simulink model "final_dynamic_24a"  (R2025a)
settings: Solver=ode15s  StartTime=0.0  StopTime=14000  RelTol=1e-3  AbsTol=1e-6
undefined symbols (not defined in the file): A_rad, bp_er, bp_mf, bp_speed, Cp_rad, epsilon, ETAT_table, h_h, M_rad, m_ratio_bp, mdot_design, paper54, PR_table, speed_bp, table_eff, table_mf, theta
libraries: simulink x4
(part 2 of 2)

== system final_dynamic_24a/rediator/Subsystem ==
  Constant : Constant  Value=epsilon
  Constant1 : Constant  Value=theta
  Constant2 : Constant  Value=A_rad
  Constant3 : Constant  Value=M_rad
  Constant4 : Constant  Value=Cp_rad
  Constant5 : Constant  Value=h_h
  epsilon : Outport
  theta : Outport  Port=2
  A_rad : Outport  Port=3
  M_rad : Outport  Port=4
  Cp_rad : Outport  Port=5
  h_h : Outport  Port=6
  wires:
  Constant3/1 -> M_rad/1
  Constant5/1 -> h_h/1
  Constant2/1 -> A_rad/1
  Constant1/1 -> theta/1
  Constant/1 -> epsilon/1
  Constant4/1 -> Cp_rad/1

== system final_dynamic_24a/TAC/Compressor/Corrected_Coordinates ==
  N_rpm : Inport
  mdot : Inport  Port=2
  P_in : Inport  Port=3
  T_in : Inport  Port=4
  CorrectedFlow : Product  Inputs=**/
  CorrectedSpeed : Product  Inputs=*/
  FlowAboveMinimum : simulink/Logic and Bit Operations/Compare To Constant  relop=>=  const=m_ratio_bp(1)  OutDataTypeStr=boolean
  FlowAboveMinimum_Assertion : Assertion
  FlowBelowMaximum : simulink/Logic and Bit Operations/Compare To Constant  relop=<=  const=m_ratio_bp(end)  OutDataTypeStr=boolean
  FlowBelowMaximum_Assertion : Assertion
  N_over_Ndesign : Gain  Gain=1/paper54.N_rpm
  P_over_Pdesign : Gain  Gain=1/paper54.compressor.Pin_Pa
  SpeedAboveMinimum : simulink/Logic and Bit Operations/Compare To Constant  relop=>=  const=speed_bp(1)  OutDataTypeStr=boolean
  SpeedAboveMinimum_Assertion : Assertion
  SpeedBelowMaximum : simulink/Logic and Bit Operations/Compare To Constant  relop=<=  const=speed_bp(end)  OutDataTypeStr=boolean
  SpeedBelowMaximum_Assertion : Assertion
  T_over_Tdesign : Gain  Gain=1/paper54.compressor.Tin_K
  mdot_over_mdesign : Gain  Gain=1/mdot_design
  sqrt_T_ratio : Math  Operator=sqrt
  speed_ratio : Outport
  flow_ratio : Outport  Port=2
  wires:
  SpeedAboveMinimum/1 -> SpeedAboveMinimum_Assertion/1
  SpeedBelowMaximum/1 -> SpeedBelowMaximum_Assertion/1
  FlowAboveMinimum/1 -> FlowAboveMinimum_Assertion/1
  FlowBelowMaximum/1 -> FlowBelowMaximum_Assertion/1
  N_rpm/1 -> N_over_Ndesign/1
  mdot/1 -> mdot_over_mdesign/1
  P_in/1 -> P_over_Pdesign/1
  T_in/1 -> T_over_Tdesign/1
  T_over_Tdesign/1 -> sqrt_T_ratio/1
  N_over_Ndesign/1 -> CorrectedSpeed/1
  sqrt_T_ratio/1 -> CorrectedSpeed/2, CorrectedFlow/2
  mdot_over_mdesign/1 -> CorrectedFlow/1
  P_over_Pdesign/1 -> CorrectedFlow/3
  CorrectedSpeed/1 -> speed_ratio/1, SpeedAboveMinimum/1, SpeedBelowMaximum/1
  CorrectedFlow/1 -> flow_ratio/1, FlowAboveMinimum/1, FlowBelowMaximum/1

== system final_dynamic_24a/TAC/Turbine/Pressure Drop ==
  2-3 : Constant  Value=0
  3-4 : Constant  Value=0.011605
  5-6 : Constant  Value=0.005158
  6-1 : Constant  Value=0.002579
  constant : Constant
  1 : Outport
  p5-6 : Outport  Port=2
  p6-1 : Outport  Port=3
  p2-3 : Outport  Port=4
  p3-4 : Outport  Port=5
  wires:
  5-6/1 -> p5-6/1
  3-4/1 -> p3-4/1
  constant/1 -> 1/1
  6-1/1 -> p6-1/1
  2-3/1 -> p2-3/1

== matlab function final_dynamic_24a/IHX/IHX_region_1/HeXe_Properties_cold ==
  data: T_c1_average input; cp output; P_in input
function cp = HeXe_Properties_cold(T_c1_average,P_in)

coder.extrinsic('HeXe_property_simulink');

cp = 0;
[cp, ~, ~, ~, ~, ~] = ...
    HeXe_property_simulink(T_c1_average, P_in);
end

== matlab function final_dynamic_24a/IHX/IHX_region_1/Lithium_Properties_hot ==
  data: T_h1_average input; P_c input; cp output
function cp = Lithium_Properties_hot(T_h1_average, P_c)
% 热侧液锂比热容。
% 为保持原有两个输入端口和连线不变，保留 P_c；
% 液锂物性使用设计压力 0.234 MPa。

coder.extrinsic('Lithium_property_simulink');

cp = 0;
[cp, ~, ~, ~, ~, ~] = ...
    Lithium_property_simulink(T_h1_average, 0.234e6);
end

== matlab function final_dynamic_24a/IHX/IHX_region_2/Lithium_Properties_hot ==
  data: T_h1_average input; P_c input; cp output
function cp = Lithium_Properties_hot(T_h1_average, P_c)
% 热侧液锂比热容。
% 为保持原有两个输入端口和连线不变，保留 P_c；
% 液锂物性使用设计压力 0.234 MPa。

coder.extrinsic('Lithium_property_simulink');

cp = 0;
[cp, ~, ~, ~, ~, ~] = ...
    Lithium_property_simulink(T_h1_average, 0.234e6);
end

== matlab function final_dynamic_24a/TAC/Compressor/HeXe_Properties (point 1) ==
  data: T_in input; P_in input; gamma output
function gamma = HeXe_Properties_hot(T_in, P_in)
coder.extrinsic('HeXe_property_simulink');
gamma=0;
[~, gamma, ~, ~, ~, ~] = HeXe_property_simulink(T_in, P_in);
end

== matlab function final_dynamic_24a/IHX/IHX_region_2/HeXe_Properties_cold ==
  data: T_c1_average input; cp output; P_in input
function cp = HeXe_Properties_cold(T_c1_average,P_in)

coder.extrinsic('HeXe_property_simulink');

cp = 0;
[cp, ~, ~, ~, ~, ~] = ...
    HeXe_property_simulink(T_c1_average, P_in);
end

== matlab function final_dynamic_24a/TAC/Compressor/HeXe_Properties(point 1)1 ==
  data: T_in input; P_in input; cp1 output
function cp1 = HeXe_Properties(T_in, P_in)
coder.extrinsic('HeXe_property_simulink');
cp1 = 0; 
[cp1, ~, ~, ~, ~, ~] = HeXe_property_simulink(T_in, P_in);
end

== matlab function final_dynamic_24a/TAC/Compressor/HeXe_Properties(point 2s) ==
  data: T5s input; P_out input; cp2 output
function cp2 = HeXe_Properties(T5s, P_out)
coder.extrinsic('HeXe_property_simulink');
cp2 = 0; 
[cp2, ~, ~, ~, ~, ~] = HeXe_property_simulink(T5s, P_out);
end

== matlab function final_dynamic_24a/TAC/Compressor/MATLAB Function ==
  data: T_in input; r input; T5s output; gamma input
function T5s = fcn(T_in, r, gamma)
T5s = T_in * r^((gamma - 1)/gamma);
end

== matlab function final_dynamic_24a/recuperator/MannRegion_1/HeXe_Properties_cold ==
  data: T_in input; P_in input; cp output
function cp = HeXe_Properties_cold(T_in, P_in)
% 调用外置函数计算 He-Xe 比热容
coder.extrinsic('HeXe_property_simulink');

cp = 0;                                     % 必须先初始化
[cp, ~, ~, ~, ~, ~] = HeXe_property_simulink(T_in, P_in);  % 调用外部文件
end

== matlab function final_dynamic_24a/recuperator/MannRegion_1/HeXe_Properties_hot ==
  data: T_in input; P_in input; cp output
function cp = HeXe_Properties_hot(T_in, P_in)
% 调用外置函数计算 He-Xe 比热容
coder.extrinsic('HeXe_property_simulink');

cp = 0;                                     % 必须先初始化
[cp, ~, ~, ~, ~, ~] = HeXe_property_simulink(T_in, P_in);  % 调用外部文件
end

== matlab function final_dynamic_24a/recuperator/MannRegion_2/HeXe_Properties_cold ==
  data: T_in input; P_in input; cp output
function cp = HeXe_Properties_cold(T_in, P_in)
% 调用外置函数计算 He-Xe 比热容
coder.extrinsic('HeXe_property_simulink');

cp = 0;                                     % 必须先初始化
[cp, ~, ~, ~, ~, ~] = HeXe_property_simulink(T_in, P_in);  % 调用外部文件
end

== matlab function final_dynamic_24a/recuperator/MannRegion_2/HeXe_Properties_hot ==
  data: T_in input; P_in input; cp output
function cp = HeXe_Properties_hot(T_in, P_in)
% 调用外置函数计算 He-Xe 比热容
coder.extrinsic('HeXe_property_simulink');

cp = 0;                                     % 必须先初始化
[cp, ~, ~, ~, ~, ~] = HeXe_property_simulink(T_in, P_in);  % 调用外部文件
end

== matlab function final_dynamic_24a/TAC/Compressor/MATLAB Function1 ==
  data: T_out output; T_in input; eta_c input; cp1 input; cp2 input; T5s input
function T_out = Fcn(T_in, eta_c, cp1, cp2, T5s)
T_out = T_in + (cp2*(T5s - T_in))/(cp1*eta_c);
end

== matlab function final_dynamic_24a/precooler/precooler_1/HeXe_Properties_hot ==
  data: T_in input; P_in input; cp output
function cp = HeXe_Properties_hot(T_in, P_in)
% 调用外置函数计算 He-Xe 比热容
coder.extrinsic('HeXe_property_simulink');

cp = 0;                                     % 必须先初始化
[cp, ~, ~, ~, ~, ~] = HeXe_property_simulink(T_in, P_in);  % 调用外部文件
end

== matlab function final_dynamic_24a/precooler/precooler_1/NaK_Properties_cold ==
  data: T_in input; cp output
function cp = NaK_Properties_cold(T_in)
cp = 1000.*(1.061 - 3.694e-4.*T_in + 4.615e-8.*T_in.^2 + 1.509e-10.*T_in.^3);
end

== matlab function final_dynamic_24a/precooler/precooler_2/HeXe_Properties_hot ==
  data: T_in input; P_in input; cp output
function cp = HeXe_Properties_hot(T_in, P_in)
% 调用外置函数计算 He-Xe 比热容
coder.extrinsic('HeXe_property_simulink');

cp = 0;                                     % 必须先初始化
[cp, ~, ~, ~, ~, ~] = HeXe_property_simulink(T_in, P_in);  % 调用外部文件
end

== matlab function final_dynamic_24a/precooler/precooler_2/NaK_Properties_cold1 ==
  data: T_in input; cp output
function cp = NaK_Properties_cold(T_in)
cp = 1000.*(1.061 - 3.694e-4.*T_in + 4.615e-8.*T_in.^2 + 1.509e-10.*T_in.^3);
end

== matlab function final_dynamic_24a/rediator/MATLAB Function ==
  data: T input; Cp output
function Cp = Cp_h(T)
Cp = 1000.*(1.061 - 3.694e-4.*T + 4.615e-8.*T.^2 + 1.509e-10.*T.^3);
end

== matlab function final_dynamic_24a/TAC/Turbine/HeXe_Properties (point 1) ==
  data: T_in input; P_in input; gamma output
function gamma = HeXe_Properties_hot(T_in, P_in)
% 调用外置函数计算 He-Xe 比热容
coder.extrinsic('HeXe_property_simulink');
gamma=0;
[~, gamma, ~, ~, ~, ~] = HeXe_property_simulink(T_in, P_in);  % 调用外部文件
end

== matlab function final_dynamic_24a/TAC/Turbine/HeXe_Properties(point 1) ==
  data: T_in input; P_in input; cp1 output
function cp1 = HeXe_Properties(T_in, P_in)
% 调用外置函数计算 He-Xe 比热容
coder.extrinsic('HeXe_property_simulink');
cp1 = 0; 
[cp1, ~, ~, ~, ~, ~] = HeXe_property_simulink(T_in, P_in);  % 调用外部文件
end

== matlab function final_dynamic_24a/TAC/Turbine/HeXe_Properties(point 2s) ==
  data: T_in input; P_in input; cp2 output
function cp2 = HeXe_Properties(T_in, P_in)
% 调用外置函数计算 He-Xe 比热容
coder.extrinsic('HeXe_property_simulink');
cp2 = 0; 
[cp2, ~, ~, ~, ~, ~] = HeXe_property_simulink(T_in, P_in);  % 调用外部文件
end

== matlab function final_dynamic_24a/TAC/Turbine/MATLAB Function ==
  data: pi input; T2s output; phi input; T1 input
function T2s = fcn(pi, phi, T1)
    T2s = T1 * pi^(-phi);
end

== matlab function final_dynamic_24a/TAC/Turbine/MATLAB Function1 ==
  data: T2 output; T1 input; neta input; cp1 input; cp2 input; T2s input
function T2= Fcn(T1,neta,cp1,cp2,T2s)
T2=T1-(neta*cp2*(T1-T2s))/cp1;
end
